simulink model "bh_explore_it"  (R2016a)
settings: Solver=ode23t  StartTime=0.0  StopTime=5  FixedStep=0.001  RelTol=1e-5
undefined symbols (not defined in the file or in its folder): P_veh
libraries: simulink_extras x3, bh_6dof_LIBRARY x2
settings Model: Creator=bhorton  LastModifiedBy=bhorton
settings DataIOCC: SaveOutput=off  SignalLogging=off  DSMLogging=off  VisualizeSimOutput=off  SaveTime=off
settings DebuggingCC: AllowSymbolicDim=off
settings ModelReferenceCC: PropagateSignalLabelsOutOfModel=off
settings GRTTargetCC: GeneratePreprocessorConditionals=Use local settings

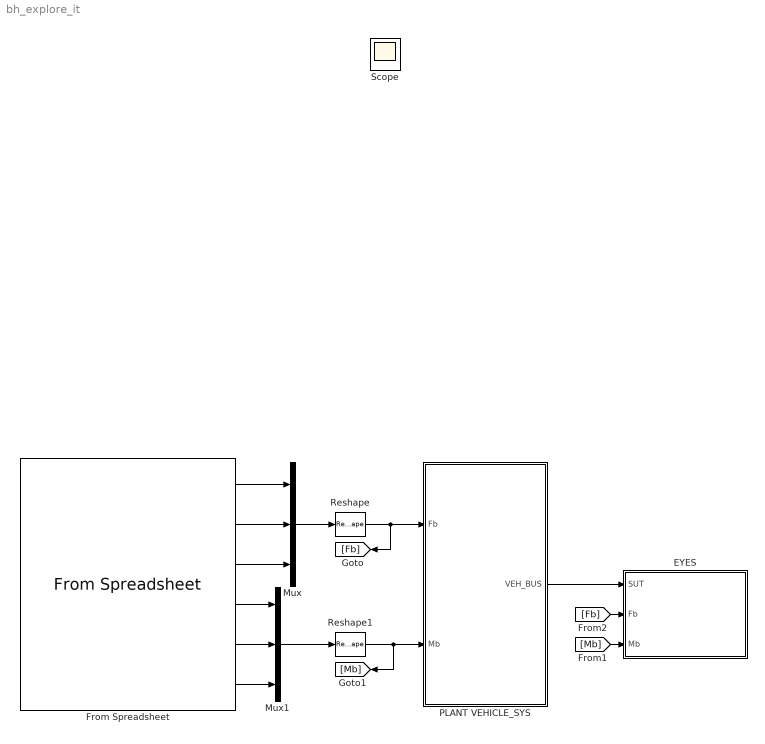
== system bh_explore_it ==
  EYES : Subsystem
      mask Display: image('bh_PIC_SCOPE.jpg');
  From Spreadsheet : FromSpreadsheet  FileName=bh_some_FbMb_TS_data.xlsx  SheetName=D_short_XYZ  ExtrapolationAfterLastDataPoint=Hold last value
  Mux : Mux  Inputs=3
  Mux1 : Mux  Inputs=3
  PLANT VEHICLE_SYS : Subsystem
  Reshape : Reshape  OutputDimensionality=Column vector (2-D)
  Reshape1 : Reshape  OutputDimensionality=Column vector (2-D)
  Scope : Scope
  wires:
  Reshape/1 -> [Fb], PLANT VEHICLE_SYS/1(Fb)
  Reshape1/1 -> [Mb], PLANT VEHICLE_SYS/2(Mb)
  PLANT VEHICLE_SYS/1(VEH_BUS) -> EYES/1(SUT)
  From Spreadsheet/1 -> Mux/1
  From Spreadsheet/2 -> Mux/2
  From Spreadsheet/3 -> Mux/3
  Mux/1 -> Reshape/1
  Mux1/1 -> Reshape1/1
  From Spreadsheet/4 -> Mux1/1
  From Spreadsheet/5 -> Mux1/2
  From Spreadsheet/6 -> Mux1/3
  [Fb] -> EYES/2(Fb)
  [Mb] -> EYES/3(Mb)

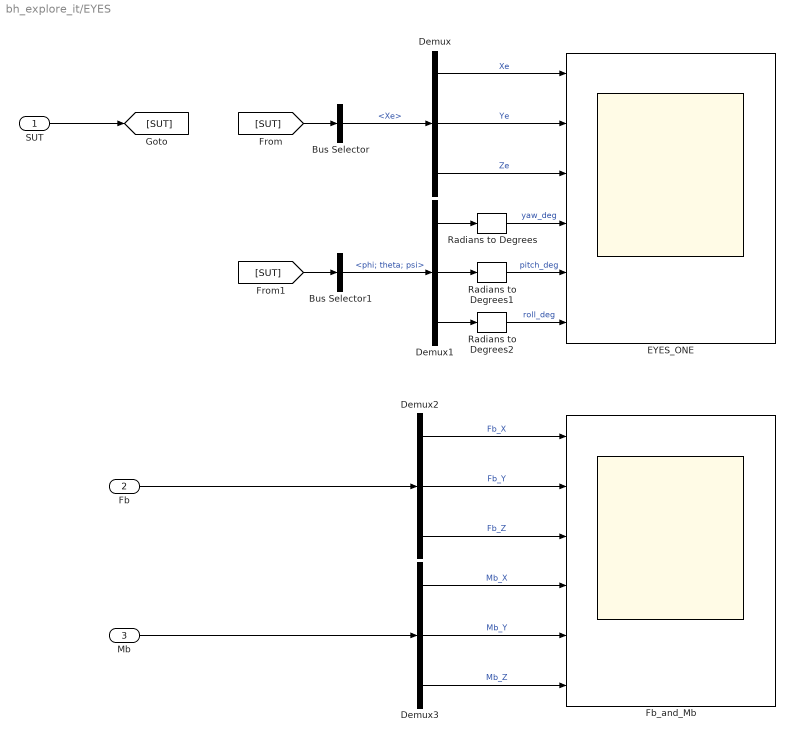
== system bh_explore_it/EYES ==
  SUT : Inport
  Fb : Inport  Port=2
  Mb : Inport  Port=3
  Bus Selector : BusSelector  OutputSignals=Xe
  Bus Selector1 : BusSelector  OutputSignals=phi; theta; psi
  Demux{,1..3} (4 alike) : Demux  Outputs=3
  EYES_ONE : Scope  NumInputPorts=6
  Fb_and_Mb : Scope  NumInputPorts=6
  Radians to Degrees : simulink_extras/Transformations/Radians to Degrees
  Radians to Degrees1 : simulink_extras/Transformations/Radians to Degrees
  Radians to Degrees2 : simulink_extras/Transformations/Radians to Degrees
  wires:
  SUT/1 -> [SUT]
  [SUT] -> Bus Selector/1
  Demux/2 -> EYES_ONE/2  "Ye"
  Demux/3 -> EYES_ONE/3  "Ze"
  Demux/1 -> EYES_ONE/1  "Xe"
  Bus Selector/1 -> Demux/1  "<Xe>"
  Bus Selector1/1 -> Demux1/1  "<phi; theta; psi>"
  [SUT] -> Bus Selector1/1
  Demux1/1 -> Radians to Degrees/1
  Radians to Degrees/1 -> EYES_ONE/4  "yaw_deg"
  Radians to Degrees1/1 -> EYES_ONE/5  "pitch_deg"
  Radians to Degrees2/1 -> EYES_ONE/6  "roll_deg"
  Demux1/3 -> Radians to Degrees2/1
  Demux1/2 -> Radians to Degrees1/1
  Fb/1 -> Demux2/1
  Demux2/1 -> Fb_and_Mb/1  "Fb_X"
  Demux2/2 -> Fb_and_Mb/2  "Fb_Y"
  Demux2/3 -> Fb_and_Mb/3  "Fb_Z"
  Mb/1 -> Demux3/1
  Demux3/1 -> Fb_and_Mb/4  "Mb_X"
  Demux3/2 -> Fb_and_Mb/5  "Mb_Y"
  Demux3/3 -> Fb_and_Mb/6  "Mb_Z"

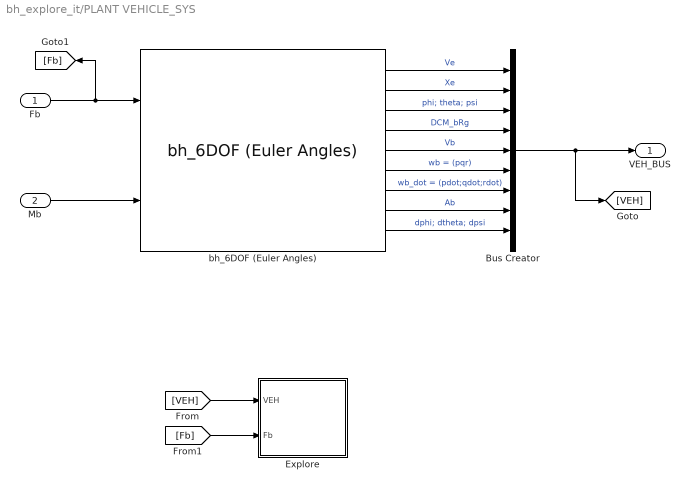
== system bh_explore_it/PLANT VEHICLE_SYS ==
  Fb : Inport
  Mb : Inport  Port=2
  Bus Creator : BusCreator  Inputs=9
  Explore : Subsystem
  bh_6DOF (Euler Angles) : bh_6dof_LIBRARY/MODELS/bh_6DOF (Euler Angles)  inertia_0=P_veh.I  mass_0=P_veh.mass  xme_0=P_veh.Xe_init  Vm_0=P_veh.Vb_init  pm_0=P_veh.wb_init  eul_0=P_veh.eul_init
  VEH_BUS : Outport
  wires:
  Fb/1 -> [Fb], bh_6DOF (Euler Angles)/1
  Mb/1 -> bh_6DOF (Euler Angles)/2
  bh_6DOF (Euler Angles)/3 -> Bus Creator/3  "phi; theta; psi"
  bh_6DOF (Euler Angles)/2 -> Bus Creator/2  "Xe"
  bh_6DOF (Euler Angles)/1 -> Bus Creator/1  "Ve"
  bh_6DOF (Euler Angles)/4 -> Bus Creator/4  "DCM_bRg"
  bh_6DOF (Euler Angles)/8 -> Bus Creator/8  "Ab"
  bh_6DOF (Euler Angles)/7 -> Bus Creator/7  "wb_dot = (pdot;qdot;rdot)"
  Bus Creator/1 -> [VEH], VEH_BUS/1
  bh_6DOF (Euler Angles)/5 -> Bus Creator/5  "Vb"
  bh_6DOF (Euler Angles)/6 -> Bus Creator/6  "wb = (pqr)"
  bh_6DOF (Euler Angles)/9 -> Bus Creator/9  "dphi; dtheta; dpsi"
  [VEH] -> Explore/1(VEH)
  [Fb] -> Explore/2(Fb)

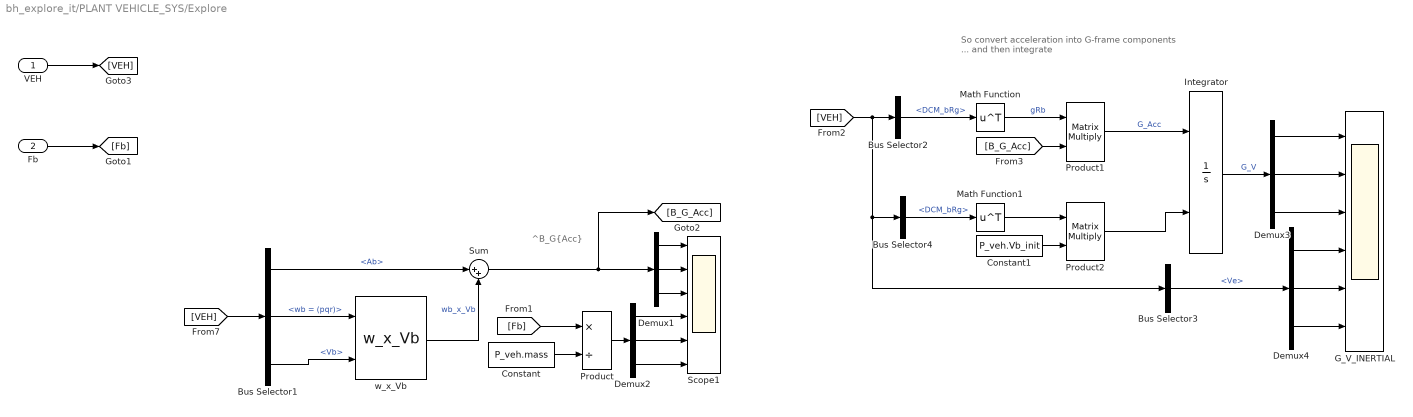
== system bh_explore_it/PLANT VEHICLE_SYS/Explore ==
  note: So convert acceleration into G-frame
      | components ... and then integrate
  note: ^B_G{Acc}
  VEH : Inport
  Fb : Inport  Port=2
  Bus Selector1 : BusSelector  OutputSignals=Ab,wb = (pqr),Vb
  Bus Selector2 : BusSelector  OutputSignals=DCM_bRg
  Bus Selector3 : BusSelector  OutputSignals=Ve
  Bus Selector4 : BusSelector  OutputSignals=DCM_bRg
  Constant : Constant  Value=P_veh.mass
  Constant1 : Constant  Value=P_veh.Vb_init
  Demux{1..4} (4 alike) : Demux  Outputs=3
  G_V_INERTIAL : Scope  NumInputPorts=6
  Integrator : Integrator  InitialConditionSource=external
  Math Function : Math  Operator=transpose  SaturateOnIntegerOverflow=on
  Math Function1 : Math  Operator=transpose  SaturateOnIntegerOverflow=on
  Product : Product  Inputs=*/
  Product1 : Product  Multiplication=Matrix(*)
  Product2 : Product  Multiplication=Matrix(*)
  Scope1 : Scope  NumInputPorts=6
  Sum : Sum  Inputs=|++
  w_x_Vb : bh_6dof_LIBRARY/MODELS/bh_6DOF (Euler Angles)/w_x_Vb  SystemSampleTime=-1
  wires:
  Demux1/1 -> Scope1/1
  [Fb] -> Product/1
  Sum/1 -> [B_G_Acc], Demux1/1
  Bus Selector1/1 -> Sum/1  "<Ab>"
  Bus Selector1/3 -> w_x_Vb/2  "<Vb>"
  Bus Selector1/2 -> w_x_Vb/1  "<wb = (pqr)>"
  Demux1/3 -> Scope1/3
  w_x_Vb/1 -> Sum/2  "wb_x_Vb"
  Demux1/2 -> Scope1/2
  Demux2/1 -> Scope1/4
  Demux2/2 -> Scope1/5
  Demux2/3 -> Scope1/6
  Fb/1 -> [Fb]
  Product/1 -> Demux2/1
  Constant/1 -> Product/2
  [VEH] -> Bus Selector4/1, Bus Selector3/1, Bus Selector2/1
  Bus Selector2/1 -> Math Function/1  "<DCM_bRg>"
  Math Function/1 -> Product1/1  "gRb"
  [B_G_Acc] -> Product1/2
  Product1/1 -> Integrator/1  "G_Acc"
  Integrator/1 -> Demux3/1  "G_V"
  Demux3/1 -> G_V_INERTIAL/1
  Demux3/2 -> G_V_INERTIAL/2
  Demux3/3 -> G_V_INERTIAL/3
  Bus Selector3/1 -> Demux4/1  "<Ve>"
  Demux4/3 -> G_V_INERTIAL/6
  Demux4/1 -> G_V_INERTIAL/4
  Demux4/2 -> G_V_INERTIAL/5
  Bus Selector4/1 -> Math Function1/1  "<DCM_bRg>"
  Math Function1/1 -> Product2/1
  Product2/1 -> Integrator/2
  Constant1/1 -> Product2/2
  [VEH] -> Bus Selector1/1
  VEH/1 -> [VEH]
